simulink model "e6"  (R2018b)
settings: Solver=VariableStepAuto  StartTime=0.0  StopTime=10.0  RelTol=1e-3
values from neighbouring files (symbols this model uses):
  B = 0.1    [e6.m]    (also in exp6.m)
  J = 0.01    [e6.m]    (also in exp6.m)
  Kb = 0.01    [e6.m]    (also in exp6.m)
  Kt = 0.01    [e6.m]    (also in exp6.m)
  R = 1    [e6.m]    (also in exp6.m)
libraries: simulink x1
settings Model: Creator=student  LastModifiedBy=hp

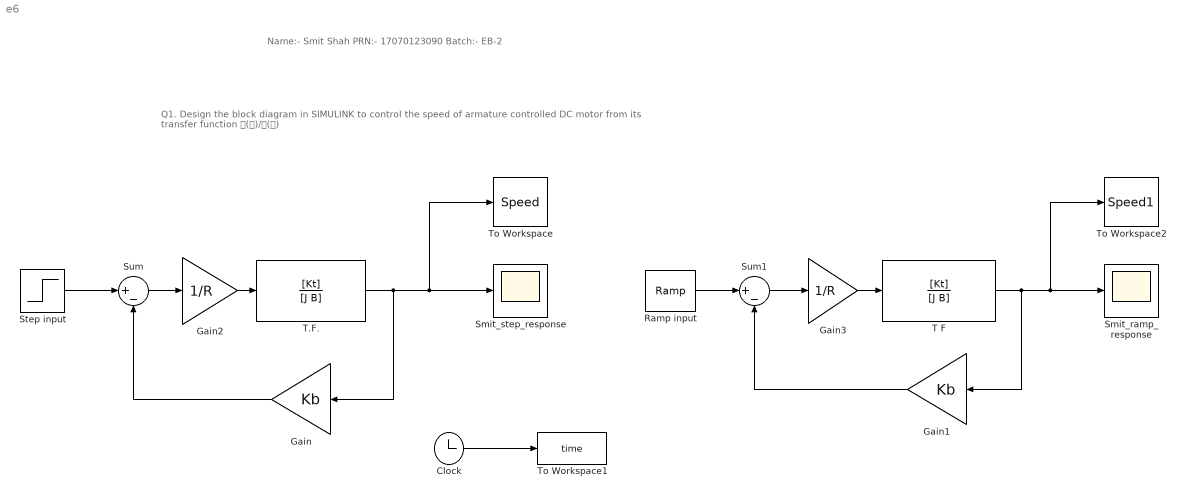
== system e6 ==
  note: Name:- Smit Shah PRN:- 17070123090 Batch:- EB-2
  note: Q1. Design the block diagram in SIMULINK to control the speed of armature controlled DC motor from its transfer function 𝜃(𝑠)/𝐸(𝑠)
  Clock : Clock
  Gain : Gain  Gain=Kb
  Gain1 : Gain  Gain=Kb
  Gain2 : Gain  Gain=1/R
  Gain3 : Gain  Gain=1/R
  Ramp input : simulink/Sources/Ramp  slope=1  start=0  InitialOutput=0
  Smit_ramp_response : Scope
  Smit_step_response : Scope
  Step input : Step  Time=0  SampleTime=0
  Sum : Sum  Inputs=|+-
  Sum1 : Sum  Inputs=|+-
  T F : TransferFcn  Numerator=[Kt]  Denominator=[J B]
  T.F. : TransferFcn  Numerator=[Kt]  Denominator=[J B]
  To Workspace : ToWorkspace  VariableName=Speed  SampleTime=-1
  To Workspace1 : ToWorkspace  VariableName=time  SampleTime=-1
  To Workspace2 : ToWorkspace  VariableName=Speed1  SampleTime=-1
  wires:
  Step input/1 -> Sum/1
  Gain/1 -> Sum/2
  T.F./1 -> Gain/1, Smit_step_response/1, To Workspace/1
  Clock/1 -> To Workspace1/1
  Ramp input/1 -> Sum1/1
  T F/1 -> Gain1/1, To Workspace2/1, Smit_ramp_response/1
  Gain1/1 -> Sum1/2
  Sum/1 -> Gain2/1
  Gain2/1 -> T.F./1
  Gain3/1 -> T F/1
  Sum1/1 -> Gain3/1
